simulink model "pmsm_model_Lab4_sensorless_st"  (R2023b)
settings: Solver=ode4  StartTime=0.0  StopTime=Tf  FixedStep=Tsim  MaxStep=Tsim  MinStep=Tsim/100  RelTol=1e-3
values from neighbouring files (symbols this model uses):
  b = 0    [pmsm_param_Lab4_2024_st.m]
  C32 = [ 1       0 ... (first row only)    [pmsm_param_Lab4_2024_st.m]
  C32inv = 2/3*[1    -1/2        -1/2 ... (first row only)    [pmsm_param_Lab4_2024_st.m]
  C33 = C32*C32inv    [pmsm_param_Lab4_2024_st.m]
  Cb = 500e-6    (= 0.0005)    [pmsm_param_Lab4_2024_st.m]
  dTm0 = Tmrated/2    (= 120)    [pmsm_param_Lab4_2024_st.m]
  Dyno = 0    [pmsm_param_Lab4_2024_st.m]
  f = 15e-3    (= 0.015)    [pmsm_param_Lab4_2024_st.m]
  frslvr = 1/Ts    (= 10000)    [pmsm_param_Lab4_2024_st.m]
  Id0 = interp1(Tref,Idopt,Tm0)    [pmsm_param_Lab4_2024_st.m]
  Idc0 = Pe0/VDC    [pmsm_param_Lab4_2024_st.m]
  Idopt = zeros(1,NT)    [pmsm_param_Lab4_2024_st.m]
  Iq0 = interp1(Tref,Iqopt,Tm0)    [pmsm_param_Lab4_2024_st.m]
  Iqopt = zeros(1,NT)    [pmsm_param_Lab4_2024_st.m]
  J = 100e-3    (= 0.1)    [pmsm_param_Lab4_2024_st.m]
  Kid = Kpd/tid    (= 180)    [pmsm_param_Lab4_2024_st.m]
  Kiq = Kpq/tiq    (= 180)    [pmsm_param_Lab4_2024_st.m]
  kL = 0.750    (= 0.75)    [pmsm_param_Lab4_2024_st.m]
  Kpd = 3*Ld0/tr    (= 3)    [pmsm_param_Lab4_2024_st.m]
  Kpll = 760    [pmsm_param_Lab4_2024_st.m]
  Kpq = 3*Lq0/tr    (= 6)    [pmsm_param_Lab4_2024_st.m]
  ksi = 0    [pmsm_param_Lab4_2024_st.m]
  Lb = 20e-6    (= 2e-05)    [pmsm_param_Lab4_2024_st.m]
  Ld0 = 1.0*Ld    (= 0.001)    [pmsm_param_Lab4_2024_st.m]
  Lq0 = 1.0*Lq    (= 0.002)    [pmsm_param_Lab4_2024_st.m]
  Pe0 = 3/2*(Vd0*Id0+Vq0*Iq0)    [pmsm_param_Lab4_2024_st.m]
  Pp = 4    [pmsm_param_Lab4_2024_st.m]
  ppll = cell2mat(ppll)    [pmsm_param_Lab4_2024_st.m]
  Psid0 = interpn(Idv,Iqv,Psidd,Id0,Iq0)    [pmsm_param_Lab4_2024_st.m]
  Psif0 = 1.0*Psif    (= 0.167)    [pmsm_param_Lab4_2024_st.m]
  Psiq0 = interpn(Idv,Iqv,Psiqq,Id0,Iq0)    [pmsm_param_Lab4_2024_st.m]
  Qbat = 72*3600    (= 259200)    [pmsm_param_Lab4_2024_st.m]
  RateTm = 10000    [pmsm_param_Lab4_2024_st.m]
  rb = 80e-3    (= 0.08)    [pmsm_param_Lab4_2024_st.m]
  Rs = 60e-3    (= 0.06)    [pmsm_param_Lab4_2024_st.m]
  Rs0 = 1.0*Rs    (= 0.06)    [pmsm_param_Lab4_2024_st.m]
  SOC0 = 0.50    (= 0.5)    [pmsm_param_Lab4_2024_st.m]
  Thetae0 = 0    [pmsm_param_Lab4_2024_st.m]
  Tm0 = (kL+f)*Wm0    (= 0)    [pmsm_param_Lab4_2024_st.m]
  Tp = 100e-6    (= 0.0001)    [pmsm_param_Lab4_2024_st.m]
  Tref = -Tmax:Tmax/100:Tmax    [pmsm_param_Lab4_2024_st.m]
  Ts = Tp    (= 0.0001)    [pmsm_param_Lab4_2024_st.m]
  Tsim = min([Tp Ts])/100    [pmsm_param_Lab4_2024_st.m]
  TSS = Tstep+0.050    (= 0.1)    [pmsm_param_Lab4_2024_st.m]
  Tstep = 0.050    (= 0.05)    [pmsm_param_Lab4_2024_st.m]
  Ud0 = Rs*Id0    (= 0)    [pmsm_param_Lab4_2024_st.m]
  Uq0 = Rs*Iq0    [pmsm_param_Lab4_2024_st.m]
  Vd0 = Ud0-Pp*Psiq0*Wm0    [pmsm_param_Lab4_2024_st.m]
  VDC = 800    [pmsm_param_Lab4_2024_st.m]
  VDC0 = 0.8*VDC    (= 640)    [pmsm_param_Lab4_2024_st.m]
  Vp = VDC/2    (= 400)    [pmsm_param_Lab4_2024_st.m]
  Vq0 = Uq0+Pp*Psid0*Wm0    [pmsm_param_Lab4_2024_st.m]
  we0 = Pp*Wm0    (= 0)    [pmsm_param_Lab4_2024_st.m]
  Wm0 = 3000*pi/30*0    (= 0)    [pmsm_param_Lab4_2024_st.m]
  zpll = cell2mat(zpll)    [pmsm_param_Lab4_2024_st.m]
undefined symbols (not defined in the file or in its folder): DiscIntNeverNeededParam, Idd, Idrop, Iqq, Isw, kpll, Psidv, Psiqv, SwLoss, Vdrop
libraries: simulink x10
(part 1 of 2)
settings Model: Creator=babak_  LastModifiedBy=babak
settings SolverCC: AlgebraicLoopSolver=LineSearch
settings DataIOCC: LimitDataPoints=on  SaveFormat=Array  SignalLoggingSaveFormat=ModelDataLogs  ReturnWorkspaceOutputs=off
settings OptimizationCC: BooleanDataType=off  ExpressionDepthLimit=2147483647  InitFltsAndDblsToZero=on  LifeSpan=inf
settings DebuggingCC: SaveWithParameterizedLinksMsg=none  UnderspecifiedInitializationDetection=Classic  MergeDetectMultiDrivingBlocksExec=none  SignalResolutionControl=TryResolveAllWithWarning  MultiTaskDSMMsg=warning  MultiTaskCondExecSysMsg=none  FcnCallInpInsideContextMsg=warning  UnconnectedInputMsg=warning  UnconnectedOutputMsg=warning  UnconnectedLineMsg=warning  StateNameClashWarn=warning  SFUnexpectedBacktrackingDiag=warning  SFNoUnconditionalDefaultTransitionDiag=warning  ArithmeticOperatorsInVariantConditions=warning
settings HardwareCC: ProdBitPerPointer=32  ProdBitPerSizeT=32  ProdBitPerPtrDiffT=32  ProdLargestAtomicFloat=None  ProdIntDivRoundTo=Undefined  ProdEndianess=Unspecified  ProdWordSize=32  ProdHWDeviceType=32-bit Generic  TargetUnknown=on
settings ModelReferenceCC: EnableRefExpFcnMdlSchedulingChecks=on  PropagateSignalLabelsOutOfModel=off
settings SFSimCC: SimUseLocalCustomCode=off  CustomCodeUndefinedFunction=UseInterfaceOnly
settings RTWCC: RTWUseLocalCustomCode=off
settings CodeAppCC: StateflowObjectComments=on
settings GRTTargetCC: TargetFcnLib=ansi_tfl_tmw.mat  TargetLangStandard=C89/C90 (ANSI)  ModelReferenceCompliant=off  CompOptLevelCompliant=off  CombineOutputUpdateFcns=off  MatFileLogging=off  GRTInterface=on
settings ConfigComp: CovMetricSettings=dw  CovSaveCumulativeToWorkspaceVar=on  CovSaveSingleToWorkspaceVar=on  CovExternalEMLEnable=off

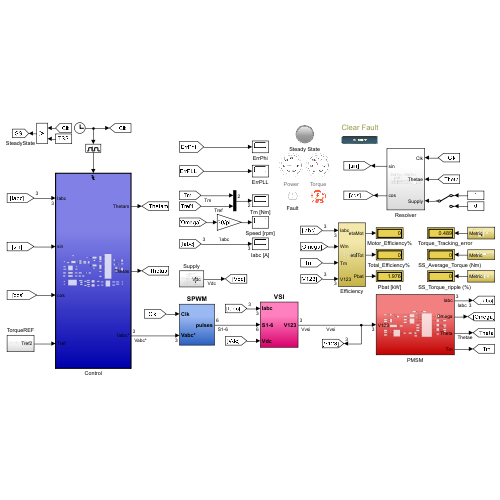
[thumbnail: Simulink's stored preview of the top-level diagram]
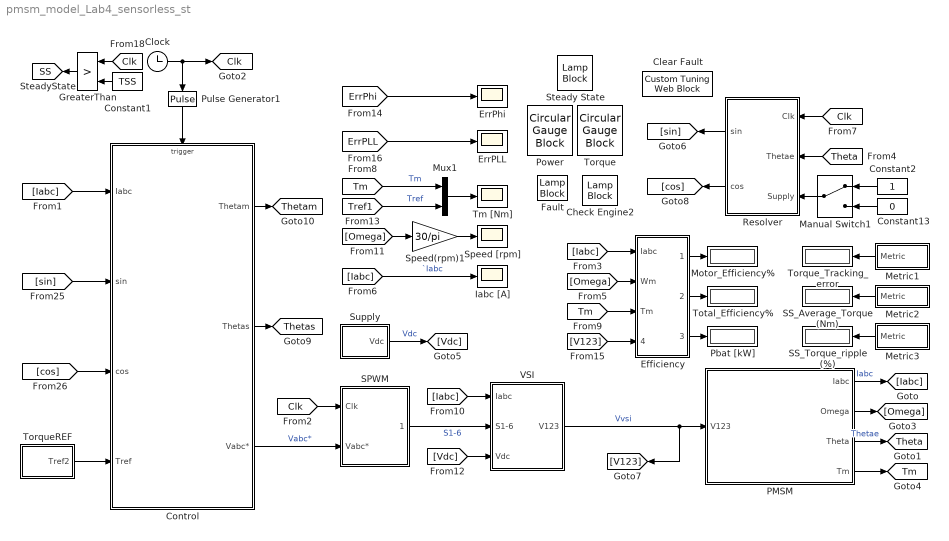
== system pmsm_model_Lab4_sensorless_st ==
  "            SS_Average_Torque (Nm)" : Display
  "      Torque_Tracking_error" : Display
  "     SS_Torque_ripple (%)" : Display
  Check Engine2 : LampBlock  LabelPosition=Hide  Icon=CheckEngine2
  Clear Fault : CustomTuningWebBlock  LabelPosition=Hide  ShowInitialText=on  Configuration="{\"components\":[{\"name\":\"BackgroundImageComponent\",\"settings\":{\"image\":{\"size\":[0,0],\"src\":\"default\",\"srcOrientation\":\"horizontal\"},\"position\":[0,0,1,1],\"scaleMode\":\"0\"}},{\"name\":\"ButtonStateComponent\",\"settings\":{\"buttonType\":\"momentary\",\"clickFcn\":\"\",\"image\":{\"size\":[180,45],\"srcOrientation\":\"Right\"},\"latched\":false,\"offValue\":[],\"onValue\":1,\"position\":[0,0,1,1],\"pressDelay\":500,\"pressFcn\":\"\",\"repeatInterval\":0,\"states\":[{\"horizontalAlignment\":\"center\",\"image\":{\"position\":[0.04444444444444445,0.005555555555555536,0.9888888888888889,0.9111111111111111],\"size\":[0.9888888888888889,0.9111111111111111],\"src\":\"data:image\\/svg+xml;base64,PHN2ZyB4bWxucz0iaHR0cDovL3d3dy53My5vcmcvMjAwMC9zdmciIHhtbG5zOnhsaW5rPSJodHRwOi8vd3d3LnczLm9yZy8xOTk5L3hsaW5rIiB2aWV3Qm94PSIwIDAgMTc3LjI1IDQwLjg4Ij48ZGVmcz48c3R5bGU+LmNscy0xe2ZpbGw6dXJsKCNyYWRpYWwtZ3JhZGllbnQpO30uY2xzLTJ7ZmlsbDp1cmwoI2xpbmVhci1ncmFkaWVudCk7fS5jbHMtM3tmaWxsOnVybCgjbGluZWFyLWdyYWRpZW50LTIpO308L3N0eWxlPjxyYWRpYWxHcmFkaWVudCBpZD0icmFkaWFsLWdyYWRpZW50IiBjeD0iOTAuMDkiIGN5PSIyMi42NiIgcj0i ...(+2212 chars)\",\"srcOrientation\":\"Right\"},\"label\":{\"color\":[1,1,0.78,1],\"icon\":{\"size\":[0.1,0.375],\"src\":\"data:image\\/svg+xml;base64,PHN2ZyBpZD0iT2ZmIiB4bWxucz0iaHR0cDovL3d3dy53My5vcmcvMjAwMC9zdmciIHhtbG5zOnhsaW5rPSJodHRwOi8vd3d3LnczLm9yZy8xOTk5L3hsaW5rIiB2aWV3Qm94PSIwIDAgNTAgNTAiPjxkZWZzPjxzdHlsZT4uY2xzLTF7ZmlsbDojN2Y4MDgwO3N0cm9rZTojMjcyNjI2O3N0cm9rZS1taXRlcmxpbWl0OjEwO3N0cm9rZS13aWR0aDozcHg7fS5jbHMtMntmaWxsOnVybCgjbGluZWFyLWdyYWRpZW50KTt9PC9zdHlsZT48bGluZWFyR3JhZGllbnQgaWQ9ImxpbmVhci1ncmFkaWVudCIgeDE9IjI1IiB5MT0iOSIgeDI9IjI1IiB5Mj0iMzciIGdyYWRpZW50VW5pdHM9InVzZXJTcGFjZU9uVXNlIj48c3RvcCBvZmZzZXQ9IjAiIHN0b3AtY29sb3I9IiNmZmYiIHN0b3Atb3BhY2l0eT0iMC43NSIvPjxzdG9wIG9mZnNldD0iMSIgc3RvcC1jb2xvcj0iI2ZmZiIgc3RvcC1vcGFjaXR5PSIwIi8+PC9saW5lYXJHcmFkaWVudD48L2RlZnM+PGNpcmNsZSBjbGFzcz0iY2xzLTEiIGN4PSIyNSIgY3k9IjI1IiByPSIyMCIvPjxjaXJjbGUgY2xhc3M9ImNscy0yIiBjeD0iMjUiIGN5PSIyMyIgcj0iMTQiLz48L3N2Zz4=\",\"srcOrientation\":\"Right\"},\"iconPlacement\":\"left\",\"opacity\":1,\"show\":true,\"text\":{\"content\":\"Button\",\"font\":\"Helvetica\",\"fontSize\":14}},\"labelOffset\":[0,0],\"verticalAlignment\":\"middle\"},{\"horizontalAlignment\":\"center\",\"image\":{\"position\":[0.04444444444444445,0.005555555555555536,0.9888888888888889,0.9111111111111111],\"size\":[0.9888888888888889,0.9111111111111111],\"src\":\"data:image\\/svg+xml;base64,PHN2ZyB4bWxucz0iaHR0cDovL3d3dy53My5vcmcvMjAwMC9zdmciIHhtbG5zOnhsaW5rPSJodHRwOi8vd3d3LnczLm9yZy8xOTk5L3hsaW5rIiB2aWV3Qm94PSIwIDAgMTc3LjI1IDQwLjg4Ij48ZGVmcz48c3R5bGU+LmNscy0xe2ZpbGw6dXJsKCNyYWRpYWwtZ3JhZGllbnQpO30uY2xzLTJ7ZmlsbDp1cmwoI2xpbmVhci1ncmFkaWVudCk7fS5jbHMtM3tmaWxsOnVybCgjbGluZWFyLWdyYWRpZW50LTIpO308L3N0eWxlPjxyYWRpYWxHcmFkaWVudCBpZD0icmFkaWFsLWdyYWRpZW50IiBjeD0iOTAuMDkiIGN5PSIyMi42NiIgcj0i ...(+2216 chars)\",\"srcOrientation\":\"Right\"},\"label\":{\"color\":[1,1,0.78,1],\"icon\":{\"size\":[0.1,0.375],\"src\":\"data:image\\/svg+xml;base64,PHN2ZyB4bWxucz0iaHR0cDovL3d3dy53My5vcmcvMjAwMC9zdmciIHhtbG5zOnhsaW5rPSJodHRwOi8vd3d3LnczLm9yZy8xOTk5L3hsaW5rIiB2aWV3Qm94PSIwIDAgNTAgNTAiPjxkZWZzPjxzdHlsZT4uY2xzLTF7ZmlsbDojNmFiZDQ1O3N0cm9rZTojMjcyNjI2O3N0cm9rZS1taXRlcmxpbWl0OjEwO3N0cm9rZS13aWR0aDozcHg7fS5jbHMtMntmaWxsOnVybCgjbGluZWFyLWdyYWRpZW50KTt9PC9zdHlsZT48bGluZWFyR3JhZGllbnQgaWQ9ImxpbmVhci1ncmFkaWVudCIgeDE9IjI1IiB5MT0iOSIgeDI9IjI1IiB5Mj0iMzciIGdyYWRpZW50VW5pdHM9InVzZXJTcGFjZU9uVXNlIj48c3RvcCBvZmZzZXQ9IjAiIHN0b3AtY29sb3I9IiNmZmYiIHN0b3Atb3BhY2l0eT0iMC43NSIvPjxzdG9wIG9mZnNldD0iMSIgc3RvcC1jb2xvcj0iI2ZmZiIgc3RvcC1vcGFjaXR5PSIwIi8+PC9saW5lYXJHcmFkaWVudD48L2RlZnM+PGcgaWQ9Ik9uIj48Y2lyY2xlIGNsYXNzPSJjbHMtMSIgY3g9IjI1IiBjeT0iMjUiIHI9IjIwIi8+PGNpcmNsZSBjbGFzcz0iY2xzLTIiIGN4PSIyNSIgY3k9IjIzIiByPSIxNCIvPjwvZz48L3N2Zz4=\",\"srcOrientation\":\"Right\"},\"iconPlacement\":\"left\",\"opacity\":1,\"show\":true,\"text\":{\"content\":\"Button\",\"font\":\"Helvetica\",\"fontSize\":14}},\"labelOffset\":[0.025,0],\"verticalAlignment\":\"middle\"},{\"horizontalAlignment\":\"center\",\"image\":{\"position\":[0.04444444444444445,0.005555555555555536,0.9888888888888889,0.9111111111111111],\"size\":[0.9888888888888889,0.9111111111111111],\"src\":\"data:image\\/svg+xml;base64,PHN2ZyB4bWxucz0iaHR0cDovL3d3dy53My5vcmcvMjAwMC9zdmciIHhtbG5zOnhsaW5rPSJodHRwOi8vd3d3LnczLm9yZy8xOTk5L3hsaW5rIiB2aWV3Qm94PSIwIDAgMTc3LjI1IDQwLjg4Ij48ZGVmcz48c3R5bGU+LmNscy0xe2ZpbGw6dXJsKCNyYWRpYWwtZ3JhZGllbnQpO30uY2xzLTJ7ZmlsbDp1cmwoI2xpbmVhci1ncmFkaWVudCk7fS5jbHMtM3tmaWxsOnVybCgjbGluZWFyLWdyYWRpZW50LTIpO308L3N0eWxlPjxyYWRpYWxHcmFkaWVudCBpZD0icmFkaWFsLWdyYWRpZW50IiBjeD0iOTAuMDkiIGN5PSIyMi42NiIgcj0i ...(+2212 chars)\",\"srcOrientation\":\"Right\"},\"label\":{\"color\":[1,1,0.78,1],\"icon\":{\"size\":[0.1,0.375],\"src\":\"data:image\\/svg+xml;base64,PHN2ZyB4bWxucz0iaHR0cDovL3d3dy53My5vcmcvMjAwMC9zdmciIHhtbG5zOnhsaW5rPSJodHRwOi8vd3d3LnczLm9yZy8xOTk5L3hsaW5rIiB2aWV3Qm94PSIwIDAgNTAgNTAiPjxkZWZzPjxzdHlsZT4uY2xzLTF7ZmlsbDojNmFiZDQ1O3N0cm9rZTojMjcyNjI2O3N0cm9rZS1taXRlcmxpbWl0OjEwO3N0cm9rZS13aWR0aDozcHg7fS5jbHMtMntmaWxsOnVybCgjbGluZWFyLWdyYWRpZW50KTt9PC9zdHlsZT48bGluZWFyR3JhZGllbnQgaWQ9ImxpbmVhci1ncmFkaWVudCIgeDE9IjI1IiB5MT0iOSIgeDI9IjI1IiB5Mj0iMzciIGdyYWRpZW50VW5pdHM9InVzZXJTcGFjZU9uVXNlIj48c3RvcCBvZmZzZXQ9IjAiIHN0b3AtY29sb3I9IiNmZmYiIHN0b3Atb3BhY2l0eT0iMC43NSIvPjxzdG9wIG9mZnNldD0iMSIgc3RvcC1jb2xvcj0iI2ZmZiIgc3RvcC1vcGFjaXR5PSIwIi8+PC9saW5lYXJHcmFkaWVudD48L2RlZnM+PGcgaWQ9Ik9uIj48Y2lyY2xlIGNsYXNzPSJjbHMtMSIgY3g9IjI1IiBjeT0iMjUiIHI9IjIwIi8+PGNpcmNsZSBjbGFzcz0iY2xzLTIiIGN4PSIyNSIgY3k9IjIzIiByPSIxNCIvPjwvZz48L3N2Zz4=\",\"srcOrientation\":\"Right\"},\"iconPlacement\":\"left\",\"opacity\":1,\"show\":true,\"text\":{\"content\":\"Button\",\"font\":\"Helvetica\",\"fontSize\":14}},\"labelOffset\":[0,0],\"verticalAlignment\":\"middle\"},{\"horizontalAlignment\":\"center\",\"image\":{\"position\":[0.04444444444444445,0.005555555555555536,0.9888888888888889,0.9111111111111111],\"size\":[0.9888888888888889,0.9111111111111111],\"src\":\"data:image\\/svg+xml;base64,PHN2ZyB4bWxucz0iaHR0cDovL3d3dy53My5vcmcvMjAwMC9zdmciIHhtbG5zOnhsaW5rPSJodHRwOi8vd3d3LnczLm9yZy8xOTk5L3hsaW5rIiB2aWV3Qm94PSIwIDAgMTc3LjI1IDQwLjg4Ij48ZGVmcz48c3R5bGU+LmNscy0xe2ZpbGw6dXJsKCNyYWRpYWwtZ3JhZGllbnQpO30uY2xzLTJ7ZmlsbDp1cmwoI2xpbmVhci1ncmFkaWVudCk7fS5jbHMtM3tmaWxsOnVybCgjbGluZWFyLWdyYWRpZW50LTIpO308L3N0eWxlPjxyYWRpYWxHcmFkaWVudCBpZD0icmFkaWFsLWdyYWRpZW50IiBjeD0iOTAuMDkiIGN5PSIyMi42NiIgcj0i ...(+2216 chars)\",\"srcOrientation\":\"Right\"},\"label\":{\"color\":[1,1,0.78,1],\"icon\":{\"size\":[0.1,0.375],\"src\":\"data:image\\/svg+xml;base64,PHN2ZyBpZD0iT2ZmIiB4bWxucz0iaHR0cDovL3d3dy53My5vcmcvMjAwMC9zdmciIHhtbG5zOnhsaW5rPSJodHRwOi8vd3d3LnczLm9yZy8xOTk5L3hsaW5rIiB2aWV3Qm94PSIwIDAgNTAgNTAiPjxkZWZzPjxzdHlsZT4uY2xzLTF7ZmlsbDojN2Y4MDgwO3N0cm9rZTojMjcyNjI2O3N0cm9rZS1taXRlcmxpbWl0OjEwO3N0cm9rZS13aWR0aDozcHg7fS5jbHMtMntmaWxsOnVybCgjbGluZWFyLWdyYWRpZW50KTt9PC9zdHlsZT48bGluZWFyR3JhZGllbnQgaWQ9ImxpbmVhci1ncmFkaWVudCIgeDE9IjI1IiB5MT0iOSIgeDI9IjI1IiB5Mj0iMzciIGdyYWRpZW50VW5pdHM9InVzZXJTcGFjZU9uVXNlIj48c3RvcCBvZmZzZXQ9IjAiIHN0b3AtY29sb3I9IiNmZmYiIHN0b3Atb3BhY2l0eT0iMC43NSIvPjxzdG9wIG9mZnNldD0iMSIgc3RvcC1jb2xvcj0iI2ZmZiIgc3RvcC1vcGFjaXR5PSIwIi8+PC9saW5lYXJHcmFkaWVudD48L2RlZnM+PGNpcmNsZSBjbGFzcz0iY2xzLTEiIGN4PSIyNSIgY3k9IjI1IiByPSIyMCIvPjxjaXJjbGUgY2xhc3M9ImNscy0yIiBjeD0iMjUiIGN5PSIyMyIgcj0iMTQiLz48L3N2Zz4=\",\"srcOrientation\":\"Right\"},\"iconPlacement\":\"left\",\"opacity\":1,\"show\":true,\"text\":{\"content\":\"Button\",\"font\":\"Helvetica\",\"fontSize\":14}},\"labelOffset\":[0.025,0],\"verticalAlignment\":\"middle\"}]}},{\"name\":\"ForegroundImageComponent\",\"settings\":{\"image\":{\"size\":[0,0],\"src\":\"default\",\"srcOrientation\":\"horizontal\"},\"isForeground\":1,\"position\":[0,0,1,1],\"scaleMode\":\"0\"}}],\"settings\":{\"BindingType\":\"param\",\"aspectRatio\":3.7777777777777777,\"backgroundColor\":[0,0,0,\"1\"],\"backgroundOffset\":0,\"backgroundOpacity\":1,\"fixedAspectRatio\":\"on\",\"foregroundColor\":[252,252,196],\"showBackgroundColor\":false,\"variant\":\"push\",\"version\":\"R2023a\"},\"type\":\"Button\"}"
  Clock : Clock
  Constant1 : Constant  Value=TSS
  Constant13 : Constant  Value=0
  Constant2 : Constant
  Control : Subsystem
  Efficiency : Subsystem
  ErrPLL : Scope
  ErrPhi : Scope
  Fault : LampBlock  LabelPosition=Hide  Icon=TireMonitor
  GreaterThan : RelationalOperator  Operator=>  RndMeth=Simplest  InputSameDT=off
  Iabc [A] : Scope
  Manual Switch1 : ManualSwitch
  Metric1 : Subsystem
  Metric2 : Subsystem
  Metric3 : Subsystem
  Motor_Efficiency% : Display
  Mux1 : Mux  Inputs=2
  PMSM : Subsystem
  Pbat [kW] : Display
  Power : CircularGaugeBlock  LabelPosition=Hide  ScaleMin=-20
  Pulse Generator1 : DiscretePulseGenerator  PulseType=Time based  TimeSource=Use external signal  Period=Ts  PhaseDelay=Tsim
  Resolver : Subsystem
  SPWM : Subsystem
  Speed [rpm] : Scope
  Speed(rpm)1 : Gain  Gain=30/pi
  Steady State : LampBlock  LabelPosition=Hide
  Supply : Subsystem
      settings: PortSchema="{\"entries\":[{\"content\":{\"sides\":[{\"content\":{\"connectorIds\":[]},\"type\":\"ConnectorPlacement.EquallySpacedRectSide\",\"uuid\":\"f6a50b0e-e406-44ec-a837-188ccf25c988\"},{\"content\":{\"connectorIds\":[],\"side\":\"RIGHT\"},\"type\":\"ConnectorPlacement.EquallySpacedRectSide\",\"uuid\":\"758525d2-b429-4a35-a56f-d60ac10ca8a9\"},{\"content\":{\"connectorIds\":[\"Out1\"],\"side\":\"TOP\"},\"type\":\"ConnectorPlacement.EquallySpacedRectSide\",\"uuid\":\"bedbcc07-640a-4a94-abcb-a05396b336d1\"}]},\"type\":\"ConnectorPlacement.EquallySpacedConnector\",\"uuid\":\"fd90f98a-c249-4d99-b745-2239d5baaabe\"}],\"packageUris\":[\"http://schema.mathworks.com/mf0/Connector/R2020b\"],\"version\":\"1.0\"}"
  Tm [Nm] : Scope
  Torque : CircularGaugeBlock  LabelPosition=Hide  ScaleMax=300
  TorqueREF : Subsystem
  "Total_Efficiency% " : Display
  VSI : Subsystem
  tag scope: Clk=global, SS=global, Theta=global, Thetam=global, Thetas=global, Tm=global
  wires:
  PMSM/3(Theta) -> [Theta]  "Thetae"
  PMSM/4(Tm) -> [Tm]
  Clock/1 -> [Clk], Pulse Generator1/1
  PMSM/1(Iabc) -> [Iabc]  "Iabc"
  [Iabc] -> Control/1(Iabc)
  PMSM/2(Omega) -> [Omega]
  Supply/1("Vdc ") -> [Vdc]  "Vdc"
  SPWM/1(pulses) -> VSI/2(S1-6)  "S1-6"
  [Iabc] -> VSI/1(Iabc)
  [Clk] -> SPWM/1(Clk)
  VSI/1(V123) -> PMSM/1(V123), [V123]  "Vvsi"
  [Iabc] -> Efficiency/1(Iabc)
  Efficiency/1(etaMot) -> Motor_Efficiency%/1
  [Tm] -> Efficiency/3(Tm)
  [Omega] -> Efficiency/2(Wm)
  Efficiency/2(etaTot) -> "Total_Efficiency% "/1
  Metric1/1("Metric ") -> "      Torque_Tracking_error"/1
  Metric2/1(Metric) -> "            SS_Average_Torque (Nm)"/1
  Metric3/1(Metric) -> "     SS_Torque_ripple (%)"/1
  Speed(rpm)1/1 -> Speed [rpm]/1
  [Omega] -> Speed(rpm)1/1
  [Clk] -> GreaterThan/1
  [Iabc] -> Iabc [A]/1  "`Iabc"
  Constant1/1 -> GreaterThan/2
  GreaterThan/1 -> [SS]
  Control/3(Vabc*) -> SPWM/2(Vabc*)  "Vabc*"
  [Vdc] -> VSI/3(Vdc)
  Pulse Generator1/1 -> Control/Trigger
  Efficiency/3(Pbat) -> Pbat [kW]/1
  TorqueREF/1(Tref2) -> Control/4(Tref)
  [V123] -> Efficiency/4(V123)
  Mux1/1 -> Tm [Nm]/1
  [Tm] -> Mux1/1  "Tm"
  [Tref1] -> Mux1/2  "Tref"
  [Clk] -> Resolver/1(Clk)
  Constant13/1 -> Manual Switch1/2
  Resolver/2(cos) -> [cos]
  [Theta] -> Resolver/2(Thetae)
  Resolver/1(sin) -> [sin]
  Manual Switch1/1 -> Resolver/3(Supply)
  Constant2/1 -> Manual Switch1/1
  [sin] -> Control/2(sin)
  [cos] -> Control/3(cos)
  Control/2(Thetas) -> [Thetas]
  Control/1(Thetam) -> [Thetam]
  [ErrPhi] -> ErrPhi/1
  [ErrPLL] -> ErrPLL/1

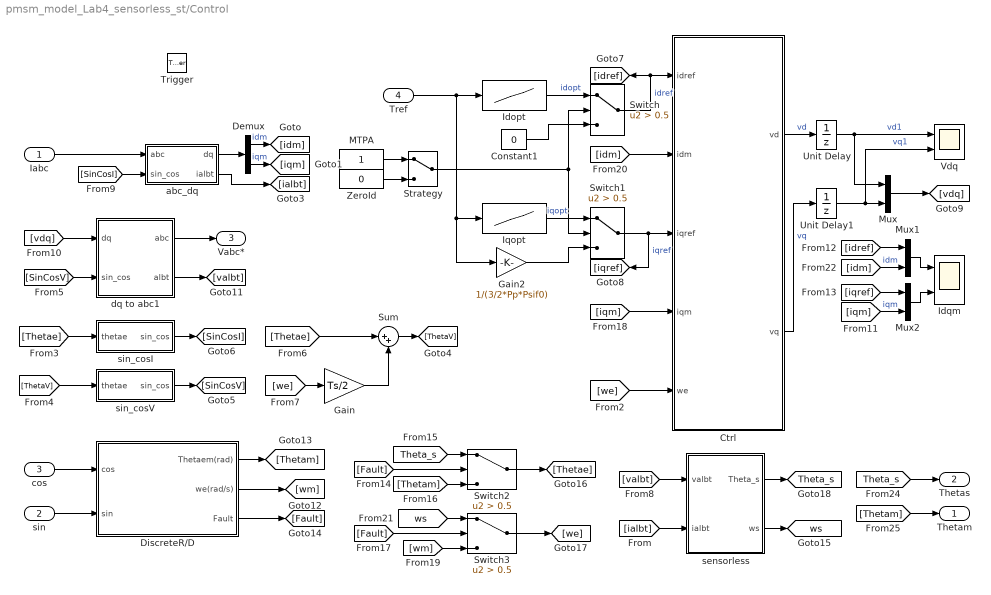
== system pmsm_model_Lab4_sensorless_st/Control ==
  Iabc : Inport
  sin : Inport  Port=2
  cos : Inport  Port=3
  Tref : Inport  Port=4
  Trigger : TriggerPort  TriggerType=falling  VariantControl=Variant  PortDimensions=1
  Constant1 : Constant  Value=0
  Ctrl : MATLAB Function  TreatAsAtomicUnit=on
  Demux : Demux  Outputs=2
  DiscreteR/D : Subsystem
  Gain : Gain  Gain=Ts/2
  Gain2 : Gain  Gain=1/(3/2*Pp*Psif0)
  Idopt : Lookup_n-D  NumberOfTableDimensions=1  BreakpointsForDimension1=Tref  Table=Idopt  InternalRulePriority=Speed  RndMeth=Simplest
  Idqm : Scope  NumInputPorts=2
  Iqopt : Lookup_n-D  NumberOfTableDimensions=1  BreakpointsForDimension1=Tref  Table=Iqopt  InternalRulePriority=Speed  RndMeth=Simplest
  MTPA : Constant
  Mux : Mux  Inputs=2
  Mux1 : Mux  Inputs=2
  Mux2 : Mux  Inputs=2
  Strategy : ManualSwitch
  Sum : Sum  Inputs=|++
  Switch{,1..3} (4 alike) : Switch  Criteria=u2 > Threshold  Threshold=0.5  SaturateOnIntegerOverflow=off  InputSameDT=off
  Unit Delay : UnitDelay  InitialCondition=Vd0  SampleTime=-1  HasFrameUpgradeWarning=on
  Unit Delay1 : UnitDelay  InitialCondition=Vq0  SampleTime=-1  HasFrameUpgradeWarning=on
  Vdq : Scope  NumInputPorts=2
  ZeroId : Constant  Value=0
  abc_dq : Subsystem
  dq to abc1 : Subsystem
  sensorless : Subsystem
  sin_cosI : Subsystem
  sin_cosV : Subsystem
  Thetam : Outport
  Thetas : Outport  Port=2
  Vabc* : Outport  Port=3
  tag scope: Theta_s=global, ws=global
  wires:
  sin_cosI/1(sin_cos) -> [SinCosI]
  Ctrl/2(vq) -> Unit Delay1/1  "vq"
  Ctrl/1(vd) -> Unit Delay/1  "vd"
  [Thetae] -> sin_cosI/1(thetae)
  [ThetaV] -> sin_cosV/1(thetae)
  sin_cosV/1(sin_cos) -> [SinCosV]
  Sum/1 -> [ThetaV]
  [Thetae] -> Sum/1
  [we] -> Gain/1
  Gain/1 -> Sum/2
  [iqm] -> Mux2/2  "iqm"
  [idm] -> Mux1/2  "idm"
  Mux2/1 -> Idqm/2
  Mux1/1 -> Idqm/1
  Mux/1 -> [vdq]
  [idref] -> Mux1/1
  [iqref] -> Mux2/1
  [idm] -> Ctrl/2(idm)
  [we] -> Ctrl/5(we)
  [iqm] -> Ctrl/4(iqm)
  Idopt/1 -> Switch/1  "idopt"
  Iqopt/1 -> Switch1/1  "iqopt"
  Tref/1 -> Gain2/1, Iqopt/1, Idopt/1
  Unit Delay/1 -> Mux/1, Vdq/1  "vd1"
  Unit Delay1/1 -> Mux/2, Vdq/2  "vq1"
  Switch/1 -> [idref], Ctrl/1(idref)  "idref"
  Switch1/1 -> [iqref], Ctrl/3(iqref)  "iqref"
  Strategy/1 -> Switch/2, Switch1/2
  Gain2/1 -> Switch1/3
  MTPA/1 -> Strategy/1
  ZeroId/1 -> Strategy/2
  Constant1/1 -> Switch/3
  [vdq] -> dq to abc1/1(dq)
  dq to abc1/1(abc) -> Vabc*/1
  [SinCosV] -> dq to abc1/2(sin_cos)
  dq to abc1/2(albt) -> [valbt]
  [Fault] -> Switch2/2
  sin/1 -> DiscreteR/D/2(sin)
  cos/1 -> DiscreteR/D/1(cos)
  sensorless/2(ws) -> [ws]
  DiscreteR/D/1(Thetaem(rad)) -> [Thetam]
  [ws] -> Switch3/1
  [Theta_s] -> Switch2/1
  DiscreteR/D/2(we(rad/s)) -> [wm]
  Switch3/1 -> [we]
  [valbt] -> sensorless/1(valbt)
  DiscreteR/D/3(Fault) -> [Fault]
  [Fault] -> Switch3/2
  [Thetam] -> Switch2/3
  Switch2/1 -> [Thetae]
  [wm] -> Switch3/3
  sensorless/1(Theta_s) -> [Theta_s]
  [ialbt] -> sensorless/2(ialbt)
  [Thetam] -> Thetam/1
  [Theta_s] -> Thetas/1
  Iabc/1 -> abc_dq/1(abc)
  Demux/1 -> [idm]  "idm"
  abc_dq/1(dq) -> Demux/1
  Demux/2 -> [iqm]  "iqm"
  [SinCosI] -> abc_dq/2(sin_cos)
  abc_dq/2(ialbt) -> [ialbt]

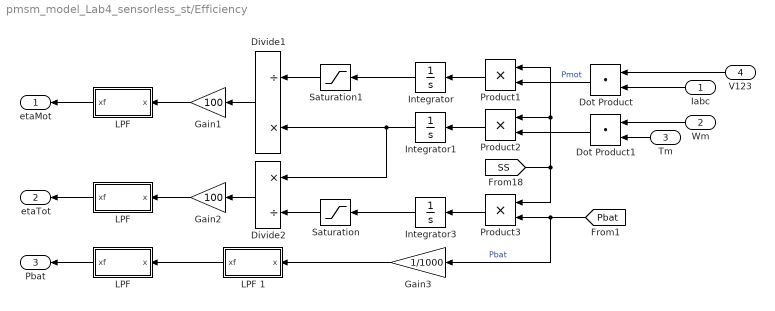
== system pmsm_model_Lab4_sensorless_st/Efficiency ==
  Iabc : Inport
  Wm : Inport  Port=2
  Tm : Inport  Port=3
  V123 : Inport  Port=4
  Divide1 : Product  Inputs=/*
  Divide2 : Product  Inputs=*/
  Dot Product : DotProduct  OutDataTypeStr=Inherit: Inherit via internal rule
  Dot Product1 : DotProduct  OutDataTypeStr=Inherit: Inherit via internal rule
  Gain1 : Gain  Gain=100
  Gain2 : Gain  Gain=100
  Gain3 : Gain  Gain=1/1000
  Integrator : Integrator  InitialCondition=1
  Integrator1 : Integrator
  Integrator3 : Integrator  InitialCondition=1
  LPF : Subsystem
  "LPF " : Subsystem
  "LPF  " : Subsystem
  LPF 1 : Subsystem
  Product1 : Product
  Product2 : Product
  Product3 : Product
  Saturation : Saturate  UpperLimit=inf  LowerLimit=1
  Saturation1 : Saturate  UpperLimit=inf  LowerLimit=1
  etaMot : Outport
  etaTot : Outport  Port=2
  Pbat : Outport  Port=3
  wires:
  Dot Product/1 -> Product1/2  "Pmot"
  Dot Product1/1 -> Product2/2
  Wm/1 -> Dot Product1/1
  V123/1 -> Dot Product/1
  Tm/1 -> Dot Product1/2
  Iabc/1 -> Dot Product/2
  Integrator1/1 -> Divide2/1, Divide1/2
  Gain1/1 -> LPF/1(x)
  Divide1/1 -> Gain1/1
  Divide2/1 -> Gain2/1
  Gain2/1 -> "LPF "/1(x)
  Saturation/1 -> Divide2/2
  [Pbat] -> Gain3/1, Product3/2  "Pbat"
  Integrator/1 -> Saturation1/1
  LPF/1(xf) -> etaMot/1
  "LPF "/1(xf) -> etaTot/1
  Integrator3/1 -> Saturation/1
  Product1/1 -> Integrator/1
  Product2/1 -> Integrator1/1
  Product3/1 -> Integrator3/1
  [SS] -> Product3/1, Product1/1, Product2/1
  Saturation1/1 -> Divide1/1
  "LPF  "/1(xf) -> Pbat/1
  Gain3/1 -> LPF 1/1(x)
  LPF 1/1(xf) -> "LPF  "/1(x)

== system pmsm_model_Lab4_sensorless_st/Metric1 ==
  Demux : Demux  Outputs=2
  ITSE : Subsystem
  LPF : Subsystem
  Multiport Switch1 : MultiPortSwitch  DataPortOrder=Zero-based contiguous  Inputs=4  zeroidx=on  SaturateOnIntegerOverflow=off  InputSameDT=off
  RMSE : Subsystem
  Sum : Sum  Inputs=+-|
  "Metric " : Outport
  wires:
  Demux/1 -> Sum/1  "Tref"
  [Tm] -> Sum/2  "Tm"
  Sum/1 -> RMSE/1(Err), ITSE/1(Err)  "Terr"
  [Tref] -> Demux/1
  Demux/2 -> Multiport Switch1/1
  Multiport Switch1/1 -> LPF/1(x)
  RMSE/1(RMSE) -> Multiport Switch1/2, Multiport Switch1/4, Multiport Switch1/5
  ITSE/1(Metric) -> Multiport Switch1/3
  LPF/1(xf) -> "Metric "/1  "Ttrack"

== system pmsm_model_Lab4_sensorless_st/Metric2 ==
  LPF : Subsystem
  Window : Subsystem
  Metric : Outport
  wires:
  Window/1(Tav) -> Metric/1  "Tav"
  [Tm] -> LPF/1(Tm)
  LPF/1(Tav) -> Window/1("Tav ")

== system pmsm_model_Lab4_sensorless_st/Metric3 ==
  Constant : Constant  Value=0
  Demux : Demux  Outputs=2
  LPF : Subsystem
  LPF2 : Subsystem
  Multiport Switch : MultiPortSwitch  DataPortOrder=Zero-based contiguous  Inputs=4  zeroidx=on  SaturateOnIntegerOverflow=off  InputSameDT=off
  Ripple : Subsystem
  Terminator : Terminator
  Metric : Outport
  wires:
  LPF/1(Tmh) -> Ripple/1(Tmh)
  [Tm] -> LPF/1(Tm)
  [Tref] -> Demux/1
  Multiport Switch/1 -> LPF2/1(x)
  Demux/2 -> Multiport Switch/1
  Demux/1 -> Terminator/1
  Constant/1 -> Multiport Switch/4, Multiport Switch/5
  Ripple/1(Ripple) -> Multiport Switch/2, Multiport Switch/3
  LPF/2(Tm0) -> Ripple/2(Tm0)
  LPF2/1(xf) -> Metric/1  "Tripple"

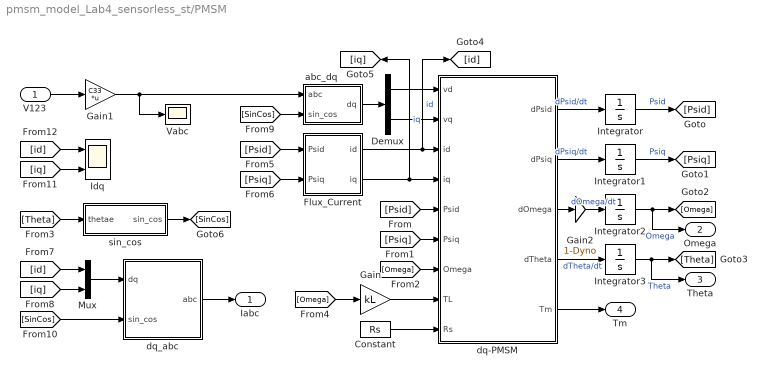
== system pmsm_model_Lab4_sensorless_st/PMSM ==
  V123 : Inport
  Constant : Constant  Value=Rs
  Demux : Demux  Outputs=2
  Flux_Current : Subsystem
  Gain : Gain  Gain=kL
  Gain1 : Gain  Gain=C33  Multiplication=Matrix(K*u)
  Gain2 : Gain  Gain=1-Dyno
  Idq : Scope  NumInputPorts=2
  Integrator : Integrator  InitialCondition=Psid0
  Integrator1 : Integrator  InitialCondition=Psiq0
  Integrator2 : Integrator  InitialCondition=Wm0
  Integrator3 : Integrator  InitialCondition=Thetae0
  Mux : Mux  Inputs=2
  Vabc : Scope
  abc_dq : Subsystem
  dq-PMSM : MATLAB Function  TreatAsAtomicUnit=on
  dq_abc : Subsystem
  sin_cos : Subsystem
  Iabc : Outport
  Omega : Outport  Port=2
  Theta : Outport  Port=3
  Tm : Outport  Port=4
  wires:
  dq-PMSM/1(dPsid) -> Integrator/1  "dPsid/dt"
  dq-PMSM/2(dPsiq) -> Integrator1/1  "dPsiq/dt"
  Integrator3/1 -> [Theta], Theta/1  "Theta"
  [Omega] -> Gain/1
  Flux_Current/1(id) -> [id], dq-PMSM/3(id)  "id"
  [SinCos] -> dq_abc/2(sin_cos)
  Integrator1/1 -> [Psiq]  "Psiq"
  sin_cos/1(sin_cos) -> [SinCos]
  dq_abc/1(abc) -> Iabc/1
  dq-PMSM/4(dTheta) -> Integrator3/1  "dTheta/dt"
  Demux/1 -> dq-PMSM/1(vd)
  [iq] -> Mux/2
  Mux/1 -> dq_abc/1(dq)
  dq-PMSM/3(dOmega) -> Gain2/1
  [Psiq] -> dq-PMSM/6(Psiq)
  [Psid] -> dq-PMSM/5(Psid)
  [Theta] -> sin_cos/1(thetae)
  abc_dq/1(dq) -> Demux/1
  [SinCos] -> abc_dq/2(sin_cos)
  Gain/1 -> dq-PMSM/8(TL)
  Demux/2 -> dq-PMSM/2(vq)
  [Omega] -> dq-PMSM/7(Omega)
  V123/1 -> Gain1/1
  [id] -> Mux/1
  Integrator2/1 -> [Omega], Omega/1  "Omega"
  Flux_Current/2(iq) -> dq-PMSM/4(iq), [iq]  "iq"
  Integrator/1 -> [Psid]  "Psid"
  Constant/1 -> dq-PMSM/9(Rs)
  Gain1/1 -> abc_dq/1(abc), Vabc/1
  dq-PMSM/5(Tm) -> Tm/1
  [id] -> Idq/1
  [iq] -> Idq/2
  [Psid] -> Flux_Current/1(Psid)
  [Psiq] -> Flux_Current/2(Psiq)
  Gain2/1 -> Integrator2/1  "dOmega/dt"

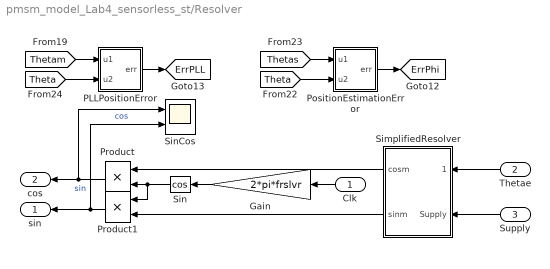
== system pmsm_model_Lab4_sensorless_st/Resolver ==
  Clk : Inport
  Thetae : Inport  Port=2
  Supply : Inport  Port=3
  Gain : Gain  Gain=2*pi*frslvr
  PLLPositionError : Subsystem
  PositionEstimationError : Subsystem
  Product : Product
  Product1 : Product
  SimplifiedResolver : Subsystem
  Sin : Trigonometry  Operator=cos
  SinCos : Scope  NumInputPorts=2
  sin : Outport
  cos : Outport  Port=2
  tag scope: ErrPLL=global, ErrPhi=global
  wires:
  SimplifiedResolver/1(cosm) -> Product/1
  SimplifiedResolver/2(sinm) -> Product1/2
  Thetae/1 -> SimplifiedResolver/1(Thetae)
  Supply/1 -> SimplifiedResolver/2(Supply)
  Product/1 -> cos/1, SinCos/1  "cos"
  Product1/1 -> sin/1, SinCos/2  "sin"
  Clk/1 -> Gain/1
  Sin/1 -> Product/2, Product1/1
  Gain/1 -> Sin/1
  [Theta] -> PositionEstimationError/2(u2)
  [Thetas] -> PositionEstimationError/1(u1)
  [Theta] -> PLLPositionError/2(u2)
  PLLPositionError/1(err) -> [ErrPLL]
  PositionEstimationError/1(err) -> [ErrPhi]
  [Thetam] -> PLLPositionError/1(u1)

== system pmsm_model_Lab4_sensorless_st/SPWM ==
  Clk : Inport
  Vabc* : Inport  Port=2
  Data Type Conversion : DataTypeConversion  SaturateOnIntegerOverflow=off  RndMeth=Floor
  Demux1 : Demux  Outputs=3
      settings: DisplayOption=none
  Mux : Mux  Inputs=6
  Relational Operator : RelationalOperator  OutDataTypeStr=boolean
  Relational Operator1 : RelationalOperator  OutDataTypeStr=boolean
  Relational Operator2 : RelationalOperator  OutDataTypeStr=boolean
  S1 : Subsystem
  S2 : Subsystem
  S3 : Subsystem
  carrier : Subsystem
  "pulses " : Scope
  pulses : Outport  InitialOutput=0
  wires:
  Mux/1 -> Data Type Conversion/1
  Clk/1 -> carrier/1(t)
  Relational Operator/1 -> S1/1("C ")
  Relational Operator1/1 -> S2/1("C ")
  Relational Operator2/1 -> S3/1("C ")
  Vabc*/1 -> Demux1/1
  Demux1/1 -> Relational Operator/1
  Demux1/2 -> Relational Operator1/1
  Demux1/3 -> Relational Operator2/1
  S1/1(C) -> Mux/1
  S1/2(C*) -> Mux/2
  S2/1(C) -> Mux/3
  S2/2(C*) -> Mux/4
  S3/1(C) -> Mux/5
  S3/2(C*) -> Mux/6
  Data Type Conversion/1 -> "pulses "/1, pulses/1
  carrier/1(Vp) -> Relational Operator2/2, Relational Operator1/2, Relational Operator/2

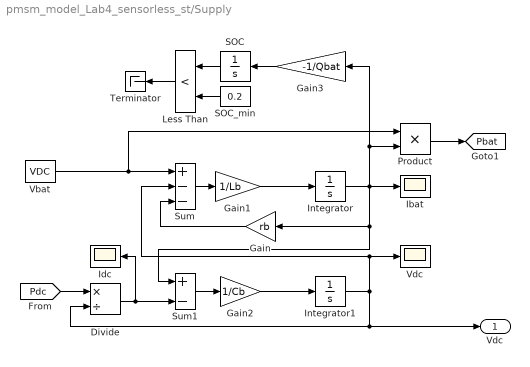
== system pmsm_model_Lab4_sensorless_st/Supply ==
  Divide : Product  Inputs=*/
  Gain : Gain  Gain=rb
  Gain1 : Gain  Gain=1/Lb
  Gain2 : Gain  Gain=1/Cb
  Gain3 : Gain  Gain=-1/Qbat
  Ibat : Scope
  Idc : Scope
  Integrator : Integrator  InitialCondition=Idc0
  Integrator1 : Integrator  InitialCondition=VDC  LimitOutput=on  LowerSaturationLimit=1
  Less Than : RelationalOperator  Operator=<  OutDataTypeStr=boolean  RndMeth=Simplest  InputSameDT=off
  Product : Product
  SOC : Integrator  InitialCondition=SOC0  LimitOutput=on  UpperSaturationLimit=1  LowerSaturationLimit=0
  SOC_min : Constant  Value=0.2
  Sum : Sum  Inputs=+--
  Sum1 : Sum  Inputs=+-
  Terminator : Terminator
  Vbat : Constant  Value=VDC
  Vdc : Scope
  "Vdc " : Outport
  tag scope: Pbat=global
  wires:
  Vbat/1 -> Sum/1, Product/1
  Integrator/1 -> Gain3/1, Product/2, Ibat/1, Gain/1, Sum1/1
  Gain1/1 -> Integrator/1
  Gain/1 -> Sum/3
  Gain2/1 -> Integrator1/1
  Sum1/1 -> Gain2/1
  Sum/1 -> Gain1/1
  Product/1 -> [Pbat]
  Divide/1 -> Idc/1, Sum1/2
  [Pdc] -> Divide/1
  Integrator1/1 -> "Vdc "/1, Divide/2, Sum/2, Vdc/1
  Gain3/1 -> SOC/1
  SOC_min/1 -> Less Than/2
  Less Than/1 -> Terminator/1
  SOC/1 -> Less Than/1

== system pmsm_model_Lab4_sensorless_st/TorqueREF ==
  Constant1 : Constant
  Delay : Delay  InitialCondition=Tm0  SampleTime=Ts
  Mux : Mux  Inputs=2
  Rate Limiter2 : RateLimiter  RisingSlewLimit=RateTm  FallingSlewLimit=-RateTm  SampleTimeMode=inherited
  Tref : Step  Time=Tstep  Before=Tm0  After=Tm0+dTm0  SampleTime=0
  Tref2 : Outport
  tag scope: Tref1=global, Tref=global
  wires:
  Delay/1 -> [Tref1], Mux/1
  Mux/1 -> [Tref]
  Tref/1 -> Rate Limiter2/1
  Rate Limiter2/1 -> Delay/1, Tref2/1
  Constant1/1 -> Mux/2

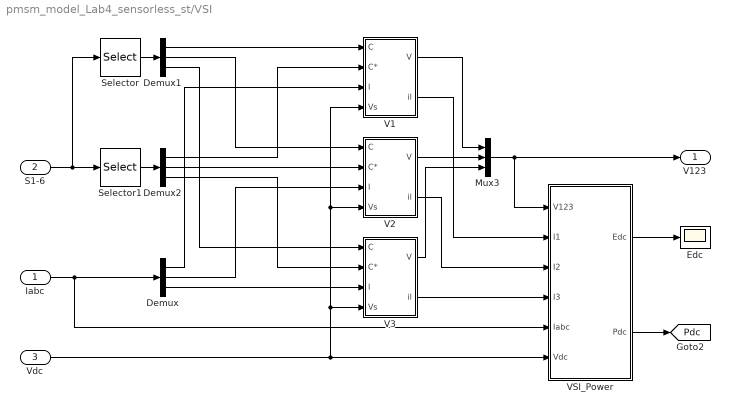
== system pmsm_model_Lab4_sensorless_st/VSI ==
  Iabc : Inport
  S1-6 : Inport  Port=2
  Vdc : Inport  Port=3
  Demux : Demux  Outputs=3
      settings: DisplayOption=none
  Demux1 : Demux  Outputs=3
      settings: DisplayOption=none
  Demux2 : Demux  Outputs=3
      settings: DisplayOption=none
  Edc : Scope
  Mux3 : Mux  Inputs=3
  Selector : Selector  InputPortWidth=6  IndexOptions=Index vector (dialog)  Indices=[1 3 5]  OutputSizes=1
  Selector1 : Selector  InputPortWidth=6  IndexOptions=Index vector (dialog)  Indices=[2 4 6]  OutputSizes=1
  V1 : Subsystem
  V2 : Subsystem
  V3 : Subsystem
  VSI_Power : Subsystem
  V123 : Outport  InitialOutput=0
  tag scope: Pdc=global
  wires:
  V3/1(V) -> Mux3/3
  V2/1(V) -> Mux3/2
  V1/1(V) -> Mux3/1
  Iabc/1 -> Demux/1, VSI_Power/5(Iabc)
  Demux/1 -> V1/3(I)
  Demux/2 -> V2/3(I)
  Demux/3 -> V3/3(I)
  Demux2/1 -> V1/2(C*)
  Demux1/1 -> V1/1(C)
  Demux1/2 -> V2/1(C)
  Demux2/2 -> V2/2(C*)
  Demux1/3 -> V3/1(C)
  Demux2/3 -> V3/2(C*)
  Mux3/1 -> V123/1, VSI_Power/1(V123)
  Vdc/1 -> V1/4(Vs), V2/4(Vs), V3/4(Vs), VSI_Power/6(Vdc)
  S1-6/1 -> Selector/1, Selector1/1
  Selector/1 -> Demux1/1
  Selector1/1 -> Demux2/1
  VSI_Power/1(Edc) -> Edc/1
  V1/2(il) -> VSI_Power/2(I1)
  V2/2(il) -> VSI_Power/3(I2)
  V3/2(il) -> VSI_Power/4(I3)
  VSI_Power/2(Pdc) -> [Pdc]

== system pmsm_model_Lab4_sensorless_st/Control/DiscreteR//D ==
  cos : Inport
  sin : Inport  Port=2
  Constant2 : Constant  Value=0
  Constant4 : Constant  Value=0
  FaultGeneration : Subsystem
  MATLAB Function : MATLAB Function  TreatAsAtomicUnit=on
  PLL : Subsystem
  Scope1 : Scope
  SinCos : Scope  NumInputPorts=2
  Thetaem(rad) : Outport
  we(rad/s) : Outport  Port=2
  Fault : Outport  Port=3
  wires:
  cos/1 -> SinCos/1, MATLAB Function/1(c), PLL/1(cos)
  sin/1 -> SinCos/2, MATLAB Function/2(s), PLL/2(sin)
  PLL/1(we(rad/s)) -> MATLAB Function/3(w), we(rad/s)/1
  PLL/2(thetae(rad)) -> Thetaem(rad)/1
  MATLAB Function/1(F) -> Scope1/1, FaultGeneration/1(F)
  Constant2/1 -> PLL/3(Reset)
  FaultGeneration/1(Fault) -> Fault/1
  Constant4/1 -> FaultGeneration/2(Clear)

== system pmsm_model_Lab4_sensorless_st/Control/abc_dq ==
  abc : Inport
  sin_cos : Inport  Port=2
  Demux : Demux  Outputs=2
      settings: DisplayOption=none
  Demux1 : Demux  Outputs=2
      settings: DisplayOption=none
  Gain3 : Gain  Gain=C32inv  Multiplication=Matrix(K*u)  OutDataTypeStr=Inherit: Same as input  ParamDataTypeStr=Inherit: Same as input
  Mux : Mux  Inputs=2
  Product{,1..3} (4 alike) : Product  InputSameDT=on  RndMeth=Zero  SaturateOnIntegerOverflow=on  OutDataTypeStr=Inherit: Same as first input
  Sum : Sum  Inputs=|++  InputSameDT=on  SaturateOnIntegerOverflow=on  OutDataTypeStr=Inherit: Same as first input
  Sum1 : Sum  Inputs=|-+  InputSameDT=on  SaturateOnIntegerOverflow=on  OutDataTypeStr=Inherit: Same as first input
  dq : Outport
  ialbt : Outport  Port=2
  wires:
  Product/1 -> Sum/1
  Product1/1 -> Sum/2
  Product2/1 -> Sum1/1
  Product3/1 -> Sum1/2
  Sum/1 -> Mux/1
  Demux/1 -> Product/1, Product2/1
  Demux1/2 -> Product/2, Product3/1
  abc/1 -> Gain3/1
  Gain3/1 -> ialbt/1, Demux/1  "alpha_beta"
  Demux/2 -> Product1/1, Product3/2
  sin_cos/1 -> Demux1/1
  Demux1/1 -> Product1/2, Product2/2
  Mux/1 -> dq/1
  Sum1/1 -> Mux/2

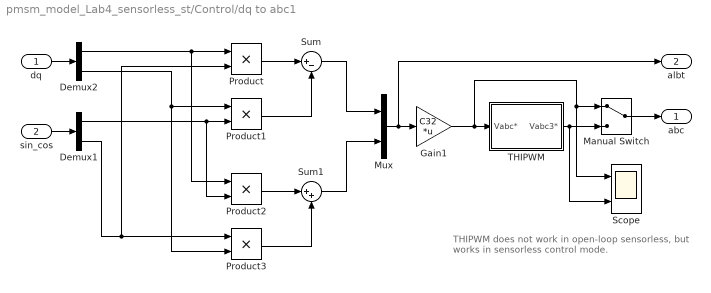
== system pmsm_model_Lab4_sensorless_st/Control/dq to abc1 ==
  note: THIPWM does not work in open-loop sensorless,
      | but works in sensorless control mode.
  dq : Inport
  sin_cos : Inport  Port=2
  Demux1 : Demux  Outputs=2
      settings: DisplayOption=none
  Demux2 : Demux  Outputs=2
      settings: DisplayOption=none
  Gain1 : Gain  Gain=C32  Multiplication=Matrix(K*u)  OutDataTypeStr=Inherit: Same as input  ParamDataTypeStr=Inherit: Same as input
  Manual Switch : ManualSwitch
  Mux : Mux  Inputs=2
  Product{,1..3} (4 alike) : Product  InputSameDT=on  RndMeth=Zero  SaturateOnIntegerOverflow=on  OutDataTypeStr=Inherit: Same as first input
  Scope : Scope  NumInputPorts=2
  Sum : Sum  Inputs=|+-  InputSameDT=on  SaturateOnIntegerOverflow=on  OutDataTypeStr=Inherit: Same as first input
  Sum1 : Sum  Inputs=|++  InputSameDT=on  SaturateOnIntegerOverflow=on  OutDataTypeStr=Inherit: Same as first input
  THIPWM : Subsystem
  abc : Outport
  albt : Outport  Port=2
  wires:
  Gain1/1 -> Scope/1, Manual Switch/1, THIPWM/1(Vabc*)
  Sum1/1 -> Mux/2
  Sum/1 -> Mux/1
  Demux2/2 -> Product1/1, Product3/2
  Demux2/1 -> Product2/1, Product/1
  Product/1 -> Sum/1
  Product1/1 -> Sum/2
  Product2/1 -> Sum1/1
  Product3/1 -> Sum1/2
  Demux1/2 -> Product/2, Product3/1
  dq/1 -> Demux2/1
  sin_cos/1 -> Demux1/1
  Demux1/1 -> Product1/2, Product2/2
  Mux/1 -> albt/1, Gain1/1
  Manual Switch/1 -> abc/1
  THIPWM/1(Vabc3*) -> Scope/2, Manual Switch/2

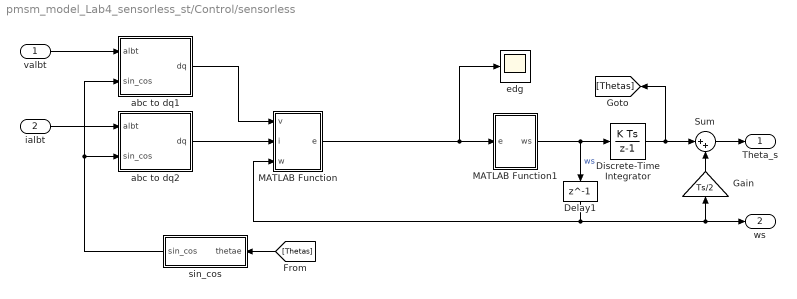
== system pmsm_model_Lab4_sensorless_st/Control/sensorless ==
  valbt : Inport
  ialbt : Inport  Port=2
  Delay1 : Delay  DelayLength=1  InitialCondition=0
  Discrete-Time Integrator : DiscreteIntegrator  gainval=1  SampleTime=-1  ICPrevOutput=DiscIntNeverNeededParam  ICPrevScaledInput=DiscIntNeverNeededParam
  Gain : Gain  Gain=Ts/2
  MATLAB Function : MATLAB Function  TreatAsAtomicUnit=on
  MATLAB Function1 : MATLAB Function  TreatAsAtomicUnit=on
  Sum : Sum  Inputs=|++
  abc to dq1 : Subsystem
  abc to dq2 : Subsystem
  edg : Scope
  sin_cos : Subsystem
  Theta_s : Outport
  ws : Outport  Port=2
  wires:
  valbt/1 -> abc to dq1/1("albt ")
  Discrete-Time Integrator/1 -> Sum/1, [Thetas]
  MATLAB Function1/1(ws) -> Delay1/1, Discrete-Time Integrator/1  "ws"
  [Thetas] -> sin_cos/1(thetae)
  sin_cos/1(sin_cos) -> abc to dq1/2(sin_cos), abc to dq2/2(sin_cos)
  abc to dq1/1(dq) -> MATLAB Function/1(v)
  Delay1/1 -> MATLAB Function/3(w), Gain/1, ws/1
  MATLAB Function/1(e) -> edg/1, MATLAB Function1/1(e)
  Sum/1 -> Theta_s/1
  Gain/1 -> Sum/2
  abc to dq2/1(dq) -> MATLAB Function/2(i)
  ialbt/1 -> abc to dq2/1("albt ")

== system pmsm_model_Lab4_sensorless_st/Control/sin_cosI ==
  thetae : Inport
  Mux1 : Mux  Inputs=2
  Trigonometric Function : Trigonometry
  Trigonometric Function1 : Trigonometry  Operator=cos
  sin_cos : Outport
  wires:
  Mux1/1 -> sin_cos/1
  thetae/1 -> Trigonometric Function/1, Trigonometric Function1/1
  Trigonometric Function1/1 -> Mux1/2
  Trigonometric Function/1 -> Mux1/1

== system pmsm_model_Lab4_sensorless_st/Control/sin_cosV ==
  thetae : Inport
  Mux1 : Mux  Inputs=2
  Trigonometric Function : Trigonometry
  Trigonometric Function1 : Trigonometry  Operator=cos
  sin_cos : Outport
  wires:
  Mux1/1 -> sin_cos/1
  thetae/1 -> Trigonometric Function/1, Trigonometric Function1/1
  Trigonometric Function1/1 -> Mux1/2
  Trigonometric Function/1 -> Mux1/1

== system pmsm_model_Lab4_sensorless_st/Efficiency/LPF ==
  x : Inport
  Gain2 : Gain  Gain=2*pi*100
  Integrator1 : Integrator
  Sum : Sum  Inputs=+-
  xf : Outport
  wires:
  Integrator1/1 -> xf/1, Sum/2
  Sum/1 -> Gain2/1
  x/1 -> Sum/1
  Gain2/1 -> Integrator1/1

== system pmsm_model_Lab4_sensorless_st/Efficiency/LPF  ==
  x : Inport
  Gain2 : Gain  Gain=2*pi*100
  Integrator1 : Integrator
  Sum : Sum  Inputs=+-
  xf : Outport
  wires:
  Gain2/1 -> Integrator1/1
  x/1 -> Sum/1
  Sum/1 -> Gain2/1
  Integrator1/1 -> xf/1, Sum/2

== system pmsm_model_Lab4_sensorless_st/Efficiency/LPF   ==
  x : Inport
  Gain2 : Gain  Gain=2*pi*10
  Integrator1 : Integrator  InitialCondition=Pe0/1000
  Sum : Sum  Inputs=+-
  xf : Outport
  wires:
  Integrator1/1 -> xf/1, Sum/2
  Sum/1 -> Gain2/1
  x/1 -> Sum/1
  Gain2/1 -> Integrator1/1

== system pmsm_model_Lab4_sensorless_st/Efficiency/LPF 1 ==
  x : Inport
  Gain2 : Gain  Gain=2*pi*3000
  Integrator1 : Integrator  InitialCondition=Pe0/1000
  Sum : Sum  Inputs=+-
  xf : Outport
  wires:
  Integrator1/1 -> Sum/2, xf/1
  Sum/1 -> Gain2/1
  x/1 -> Sum/1
  Gain2/1 -> Integrator1/1

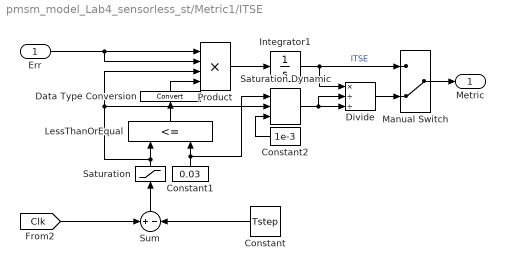
== system pmsm_model_Lab4_sensorless_st/Metric1/ITSE ==
  Err : Inport
  Constant : Constant  Value=Tstep
  Constant1 : Constant  Value=0.03
  Constant2 : Constant  Value=1e-3
  Data Type Conversion : DataTypeConversion  SaturateOnIntegerOverflow=off  RndMeth=Floor
  Divide : Product  Inputs=*//
  Integrator1 : Integrator
  LessThanOrEqual : RelationalOperator  Operator=<=  OutDataTypeStr=boolean  RndMeth=Simplest  InputSameDT=off
  Manual Switch : ManualSwitch  CurrentSetting=0
  Product : Product  Inputs=4
  Saturation : Saturate  UpperLimit=inf  LowerLimit=0
  Saturation Dynamic : simulink/Discontinuities/Saturation Dynamic  OutMin=[]  OutMax=[]  OutDataTypeStr=Inherit: Same as second input  OutDataType=fixdt(1, 16)  OutScaling=2^-10  DoSatur=off
  Sum : Sum  Inputs=+|-
  Metric : Outport
  wires:
  Sum/1 -> Saturation/1
  Integrator1/1 -> Divide/1, Manual Switch/1  "ITSE"
  Err/1 -> Product/1, Product/2
  Product/1 -> Integrator1/1
  [Clk] -> Sum/1
  Saturation/1 -> Saturation Dynamic/2, Product/3, LessThanOrEqual/1
  Constant/1 -> Sum/2
  Divide/1 -> Manual Switch/2
  Manual Switch/1 -> Metric/1
  Saturation Dynamic/1 -> Divide/3, Divide/2
  LessThanOrEqual/1 -> Data Type Conversion/1
  Constant1/1 -> Saturation Dynamic/1, LessThanOrEqual/2
  Data Type Conversion/1 -> Product/4
  Constant2/1 -> Saturation Dynamic/3

== system pmsm_model_Lab4_sensorless_st/Metric1/LPF ==
  x : Inport
  Gain : Gain  Gain=2*pi*10
  Integrator : Integrator
  Sum : Sum  Inputs=|+-
  xf : Outport
  wires:
  Gain/1 -> Integrator/1
  Sum/1 -> Gain/1
  Integrator/1 -> Sum/2, xf/1
  x/1 -> Sum/1

== system pmsm_model_Lab4_sensorless_st/Metric1/RMSE ==
  Err : Inport
  Divide : Product  Inputs=*/
  Integrator1 : Integrator
  Integrator2 : Integrator
  Product : Product  Inputs=3
  Saturation : Saturate  UpperLimit=inf  LowerLimit=1e-3
  Sqrt : Sqrt
  Sqrt1 : Sqrt
  RMSE : Outport
  wires:
  Err/1 -> Product/1, Product/2
  Product/1 -> Integrator1/1
  Integrator1/1 -> Sqrt/1
  Sqrt/1 -> Divide/1
  [SS] -> Product/3, Integrator2/1
  Divide/1 -> RMSE/1
  Integrator2/1 -> Saturation/1
  Saturation/1 -> Sqrt1/1
  Sqrt1/1 -> Divide/2

== system pmsm_model_Lab4_sensorless_st/Metric2/LPF ==
  Tm : Inport
  Gain : Gain  Gain=2*pi*10
  Integrator : Integrator  InitialCondition=Tm0
  Sum : Sum  Inputs=|+-
  Tav : Outport
  wires:
  Gain/1 -> Integrator/1
  Integrator/1 -> Tav/1, Sum/2
  Sum/1 -> Gain/1
  Tm/1 -> Sum/1

== system pmsm_model_Lab4_sensorless_st/Metric2/Window ==
  "Tav " : Inport
  Dead Zone : DeadZone  LowerValue=-inf  UpperValue=Tstep
  Manual Switch : ManualSwitch
  Product : Product
  Tav : Outport
  wires:
  [SS] -> Manual Switch/1
  Dead Zone/1 -> Manual Switch/2  "ITSE"
  Manual Switch/1 -> Product/2
  Product/1 -> Tav/1
  [Clk] -> Dead Zone/1
  "Tav "/1 -> Product/1

== system pmsm_model_Lab4_sensorless_st/Metric3/LPF ==
  Tm : Inport
  Gain : Gain  Gain=2*pi*30
  Integrator : Integrator  InitialCondition=Tm0
  Sum : Sum  Inputs=|+-
  Sum1 : Sum  Inputs=+-|
  Tmh : Outport
  Tm0 : Outport  Port=2
  wires:
  Tm/1 -> Sum1/1, Sum/1
  Integrator/1 -> Sum1/2, Tm0/1, Sum/2
  Sum/1 -> Gain/1
  Sum1/1 -> Tmh/1
  Gain/1 -> Integrator/1

== system pmsm_model_Lab4_sensorless_st/Metric3/LPF2 ==
  x : Inport
  Gain : Gain  Gain=2*pi*10
  Integrator : Integrator
  Sum : Sum  Inputs=|+-
  xf : Outport
  wires:
  Gain/1 -> Integrator/1
  Sum/1 -> Gain/1
  Integrator/1 -> Sum/2, xf/1
  x/1 -> Sum/1

== system pmsm_model_Lab4_sensorless_st/Metric3/Ripple ==
  Tmh : Inport
  Tm0 : Inport  Port=2
  Divide : Product  Inputs=*//
  Gain : Gain  Gain=100
  Integrator1 : Integrator
  Integrator2 : Integrator
  Product : Product  Inputs=3
  Saturation : Saturate  UpperLimit=inf  LowerLimit=1e-3
  Saturation1 : Saturate  UpperLimit=inf  LowerLimit=1e-3
  Sqrt : Sqrt
  Sqrt1 : Sqrt
  Ripple : Outport
  wires:
  Product/1 -> Integrator1/1
  Integrator1/1 -> Sqrt/1
  Sqrt/1 -> Divide/1
  [SS] -> Integrator2/1, Product/3
  Divide/1 -> Gain/1
  Gain/1 -> Ripple/1
  Integrator2/1 -> Saturation/1
  Saturation/1 -> Sqrt1/1
  Tm0/1 -> Saturation1/1
  Saturation1/1 -> Divide/3
  Sqrt1/1 -> Divide/2
  Tmh/1 -> Product/1, Product/2
